simulink model "long_model72423"  (R2023a)
settings: Solver=VariableStepAuto  StartTime=0.0  StopTime=600  RelTol=1e-3
undefined symbols (not defined in the file or in its folder): A_f, brakeTime, breakStrength, C_alpha, C_d, C_rr, C_s, eta_t, g, headWind, headWindTime, I_w, Im, k, l_f, l_r, lambda_f, lambda_t, M, Meq, motorDecrease, motorDecreaseTime, motorIncrease, motorIncreaseTime, motorStart, motorStartTime, mu, R_w, rho, roadSlopeTime, Vstart
libraries: simulink x1
settings Model: Creator=Samsung  LastModifiedBy=brianlesko
settings SolverCC: AlgebraicLoopSolver=TrustRegion
settings DataIOCC: ReturnWorkspaceOutputs=off
settings OptimizationCC: ReuseModelBlockBuffer=off
settings DebuggingCC: UnconnectedInputMsg=warning  UnconnectedOutputMsg=warning  UnconnectedLineMsg=warning  ArithmeticOperatorsInVariantConditions=warning
settings ModelReferenceCC: EnableRefExpFcnMdlSchedulingChecks=on
settings SFSimCC: SimUseLocalCustomCode=off  CustomCodeUndefinedFunction=UseInterfaceOnly
settings RTWCC: RTWUseLocalCustomCode=off
settings CodeAppCC: StateflowObjectComments=on

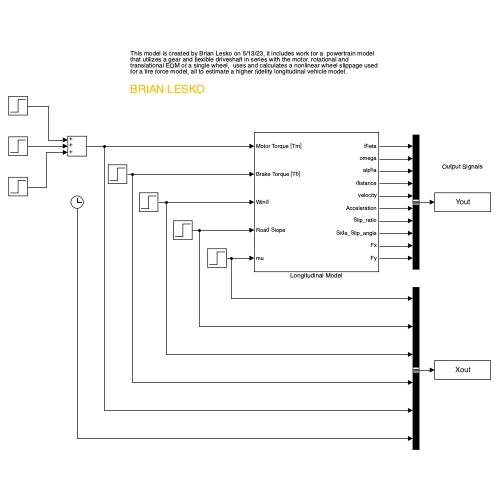
[thumbnail: Simulink's stored preview of the top-level diagram]
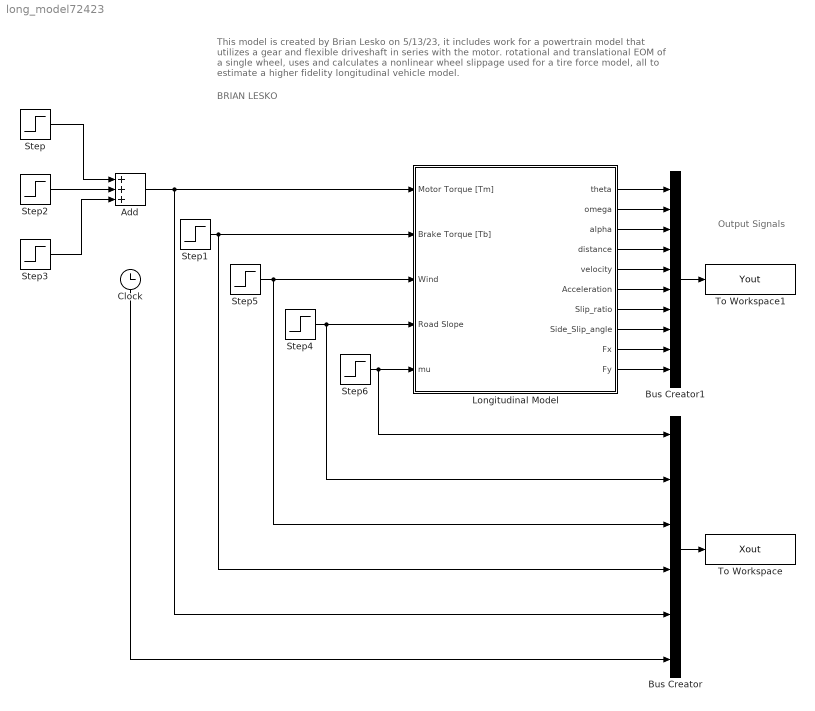
== system long_model72423 ==
  note: BRIAN LESKO
  note: This model is created by Brian Lesko on 5/13/23, it includes work for a powertrain model that utilizes a gear and flexible driveshaft in series with the motor. rotational and translational EOM of a single wheel, uses and calculates a nonlinear wheel slippage used for a tire force model, all to estimate a higher fidelity longitudinal vehicle model.
  note: Output Signals
  Add : Sum  Inputs=+++
  Bus Creator : BusCreator  Inputs=6
  Bus Creator1 : BusCreator  Inputs=10
  Clock : Clock
  Longitudinal Model : Subsystem
  Step : Step  Time=motorStartTime  After=motorStart  SampleTime=0
  Step1 : Step  Time=brakeTime  After=breakStrength  SampleTime=0
  Step2 : Step  Time=motorIncreaseTime  After=motorIncrease  SampleTime=0
  Step3 : Step  Time=motorDecreaseTime  After=-motorDecrease  SampleTime=0
  Step4 : Step  Time=roadSlopeTime  After=roadSlopeTime  SampleTime=0
  Step5 : Step  Time=headWindTime  After=headWind  SampleTime=0
  Step6 : Step  Time=0  Before=mu  After=mu  SampleTime=0
  To Workspace : ToWorkspace  VariableName=Xout  SampleTime=-1
  To Workspace1 : ToWorkspace  VariableName=Yout  SampleTime=-1
  wires:
  Step1/1 -> Longitudinal Model/2(Brake Torque [Tb]), Bus Creator/4
  Add/1 -> Bus Creator/5, Longitudinal Model/1(Motor Torque [Tm])
  Step2/1 -> Add/2
  Step3/1 -> Add/3
  Step/1 -> Add/1
  Step5/1 -> Bus Creator/3, Longitudinal Model/3(Wind)
  Step4/1 -> Bus Creator/2, Longitudinal Model/4(Road Slope)
  Step6/1 -> Bus Creator/1, Longitudinal Model/5(mu)
  Bus Creator/1 -> To Workspace/1
  Clock/1 -> Bus Creator/6
  Longitudinal Model/1(theta) -> Bus Creator1/1
  Longitudinal Model/2(omega) -> Bus Creator1/2
  Longitudinal Model/3(alpha) -> Bus Creator1/3
  Longitudinal Model/4(distance) -> Bus Creator1/4
  Longitudinal Model/5(velocity) -> Bus Creator1/5
  Longitudinal Model/6(Acceleration) -> Bus Creator1/6
  Longitudinal Model/7(Slip_ratio) -> Bus Creator1/7
  Longitudinal Model/8(Side_Slip_angle) -> Bus Creator1/8
  Longitudinal Model/9(Fx) -> Bus Creator1/9
  Longitudinal Model/10(Fy) -> Bus Creator1/10
  Bus Creator1/1 -> To Workspace1/1

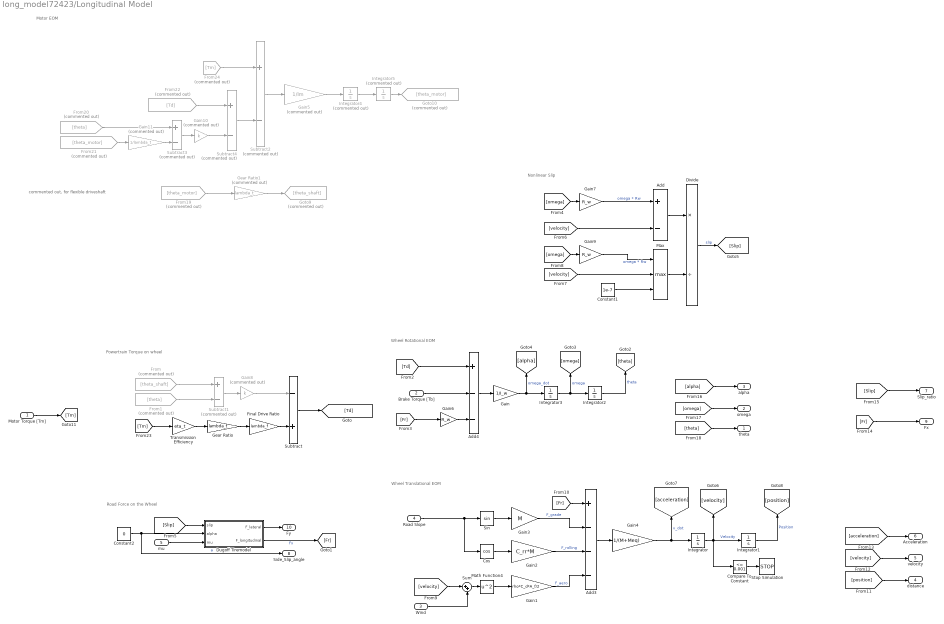
== system long_model72423/Longitudinal Model ==
  note: commented out, for flexible driveshaft
  note: Motor EOM
  note: Road Force on the Wheel
  note: Wheel Translational EOM
  note: Nonlinear Slip
  note: Wheel Rotational EOM
  note: Powertrain Torque on wheel
  Motor Torque [Tm] : Inport
  Brake Torque [Tb] : Inport  Port=2
  Wind : Inport  Port=3
  Road Slope : Inport  Port=4
  mu : Inport  Port=5
  Add : Sum  Inputs=+-
  Add3 : Sum  Inputs=+---
  Add4 : Sum  Inputs=+--
  Compare To Constant : simulink/Logic and Bit Operations/Compare To Constant  relop=<=  const=0.001  OutDataTypeStr=boolean
  Constant1 : Constant  Value=1e-7
  Constant2 : Constant  Value=0
  Cos : Trigonometry  Operator=cos
  Divide : Product  Inputs=*/
  Dugoff Tiremodel : Subsystem
  Final Drive Ratio : Gain  Gain=lambda_f
  From : From  Commented=on  GotoTag=theta_shaft
  From1 : From  Commented=on  GotoTag=theta
  From19 : From  Commented=on  GotoTag=theta_motor
  From20 : From  Commented=on  GotoTag=theta
  From21 : From  Commented=on  GotoTag=theta_motor
  From22 : From  Commented=on  GotoTag=Td
  From24 : From  Commented=on  GotoTag=Tm
  Gain : Gain  Gain=1/I_w
  Gain1 : Gain  Gain=rho*C_d*A_f/2
  Gain10 : Gain  Commented=on  Gain=k
  Gain11 : Gain  Commented=on  Gain=1/lambda_t
  Gain2 : Gain  Gain=C_rr*M
  Gain3 : Gain  Gain=M
  Gain4 : Gain  Gain=1/(M+Meq)
  Gain5 : Gain  Commented=on  Gain=1/Im
  Gain6 : Gain  Gain=R_w
  Gain7 : Gain  Gain=R_w
  Gain8 : Gain  Commented=on  Gain=k
  Gain9 : Gain  Gain=R_w
  Gear Ratio : Gain  Gain=lambda_t
  Gear Ratio1 : Gain  Commented=on  Gain=lambda_t
  Goto10 : Goto  Commented=on  GotoTag=theta_motor
  Goto9 : Goto  Commented=on  GotoTag=theta_shaft
  Integrator : Integrator  InitialCondition=Vstart  LimitOutput=on  LowerSaturationLimit=0
  Integrator1 : Integrator
  Integrator2 : Integrator  InitialCondition=1
  Integrator3 : Integrator  InitialCondition=1
  Integrator4 : Integrator  Commented=on  InitialCondition=1
  Integrator5 : Integrator  Commented=on  InitialCondition=1
  Math Function4 : Math  Operator=square  SignedPower=on
  Max : MinMax  Function=max  Inputs=3
  Sin : Trigonometry
  Stop Simulation : Stop
  Subtract : Sum  Inputs=-+
  Subtract{1..4} (4 alike) : Sum  Commented=on  Inputs=+-
  Sum : Sum  Inputs=|++
  Transmission Efficiency : Gain  Gain=eta_t
  theta : Outport  VectorParamsAs1DForOutWhenUnconnected=off
  omega : Outport  Port=2  VectorParamsAs1DForOutWhenUnconnected=off
  alpha : Outport  Port=3  VectorParamsAs1DForOutWhenUnconnected=off
  distance : Outport  Port=4  VectorParamsAs1DForOutWhenUnconnected=off
  velocity : Outport  Port=5  VectorParamsAs1DForOutWhenUnconnected=off
  Acceleration : Outport  Port=6  VectorParamsAs1DForOutWhenUnconnected=off
  Slip_ratio : Outport  Port=7
  Side_Slip_angle : Outport  Port=8
  Fx : Outport  Port=9
  Fy : Outport  Port=10
  wires:
  Integrator/1 -> Compare To Constant/1, Integrator1/1, [velocity]  "Velocity"
  Brake Torque [Tb]/1 -> Add4/2
  Compare To Constant/1 -> Stop Simulation/1
  Road Slope/1 -> Cos/1, Sin/1
  Sin/1 -> Gain3/1
  Gain2/1 -> Add3/3  "F_rolling"
  Add3/1 -> Gain4/1
  Constant2/1 -> Side_Slip_angle/1, Dugoff Tiremodel/2(alpha)  "a"
  Wind/1 -> Sum/2
  Gain7/1 -> Add/1  "omega * Rw"
  Cos/1 -> Gain2/1
  Gear Ratio/1 -> Final Drive Ratio/1
  Constant1/1 -> Max/3
  Gain/1 -> Integrator3/1, [alpha]  "omega_dot"
  Max/1 -> Divide/2
  Gain4/1 -> Integrator/1, [acceleration]  "v_dot"
  Math Function4/1 -> Gain1/1
  Transmission Efficiency/1 -> Gear Ratio/1
  Integrator3/1 -> Integrator2/1, [omega]  "omega"
  Gain1/1 -> Add3/4  "F_aero"
  Dugoff Tiremodel/1(F_lateral) -> Fy/1
  Add4/1 -> Gain/1
  Add/1 -> Divide/1
  Gain3/1 -> Add3/2  "F_grade"
  Gain6/1 -> Add4/3
  Dugoff Tiremodel/2(F_longitudinal) -> [Fr]  "Fx"
  Sum/1 -> Math Function4/1
  mu/1 -> Dugoff Tiremodel/3(mu)
  Subtract/1 -> [Td]
  From/1 -> Subtract1/1
  From1/1 -> Subtract1/2
  Subtract1/1 -> Gain8/1
  Final Drive Ratio/1 -> Subtract/2
  Gain8/1 -> Subtract/1
  [Td] -> Add4/1
  [Fr] -> Gain6/1
  Integrator2/1 -> [theta]  "theta"
  [omega] -> Gain7/1
  Divide/1 -> [Slip]  "slip"
  [Slip] -> Dugoff Tiremodel/1(slip)
  [velocity] -> Add/2
  [velocity] -> Max/2
  [omega] -> Gain9/1
  Gain9/1 -> Max/1  "omega * Rw"
  [velocity] -> Sum/1
  [Fr] -> Add3/1
  Integrator1/1 -> [position]  "Position"
  [position] -> distance/1
  [velocity] -> velocity/1
  [acceleration] -> Acceleration/1
  [Fr] -> Fx/1
  [Slip] -> Slip_ratio/1
  [alpha] -> alpha/1
  [omega] -> omega/1
  [theta] -> theta/1
  Gear Ratio1/1 -> Goto9/1
  From19/1 -> Gear Ratio1/1
  Integrator4/1 -> Integrator5/1
  Integrator5/1 -> Goto10/1
  Gain5/1 -> Integrator4/1
  From24/1 -> Subtract2/1
  Subtract2/1 -> Gain5/1
  Subtract3/1 -> Gain10/1
  From20/1 -> Subtract3/1
  Gain11/1 -> Subtract3/2
  From21/1 -> Gain11/1
  Subtract4/1 -> Subtract2/2
  Gain10/1 -> Subtract4/2
  From22/1 -> Subtract4/1
  Motor Torque [Tm]/1 -> [Tm]
  [Tm] -> Transmission Efficiency/1

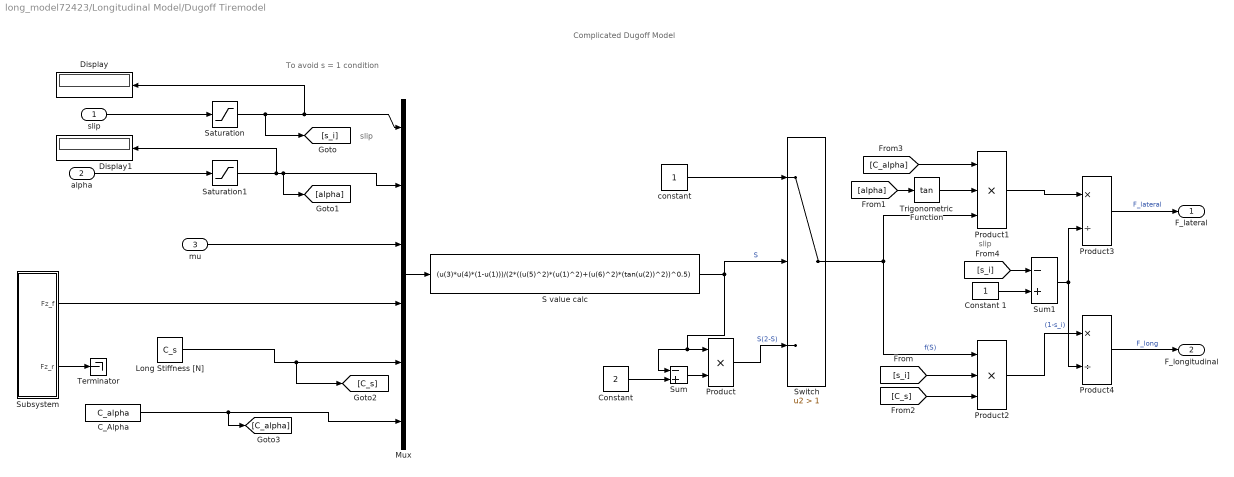
== system long_model72423/Longitudinal Model/Dugoff Tiremodel ==
  note: slip
  note: To avoid s = 1 condition
  note: Complicated Dugoff Model
  note: slip
  slip : Inport
  alpha : Inport  Port=2
  mu : Inport  Port=3
  C_Alpha : Constant  Value=C_alpha
  "Constant " : Constant  Value=2
  Constant 1 : Constant
  Display : Display
  Display1 : Display
  Long Stiffness [N] : Constant  Value=C_s
  Mux : Mux  Inputs=6
  Product : Product
  Product1 : Product  Inputs=3
  Product2 : Product  Inputs=3
  Product3 : Product  Inputs=*/
  Product4 : Product  Inputs=*/
  S value calc : Fcn  Expr=(u(3)*u(4)*(1-u(1)))/(2*((u(5)^2)*(u(1)^2)+(u(6)^2)*(tan(u(2))^2))^0.5)
  Saturation : Saturate  UpperLimit=0.999  LowerLimit=-1
  Saturation1 : Saturate  UpperLimit=20  LowerLimit=1e-4
  Subsystem : Subsystem
  Sum : Sum  Inputs=-+
  Sum1 : Sum  Inputs=-+
  Switch : Switch  Criteria=u2 > Threshold  Threshold=1  SaturateOnIntegerOverflow=off  InputSameDT=off
  Terminator : Terminator
  Trigonometric Function : Trigonometry  Operator=tan
  constant : Constant
  F_lateral : Outport  VectorParamsAs1DForOutWhenUnconnected=off
  F_longitudinal : Outport  Port=2  VectorParamsAs1DForOutWhenUnconnected=off
  wires:
  Switch/1 -> Product2/1, Product1/3  "f(S)"
  [s_i] -> Sum1/1
  Trigonometric Function/1 -> Product1/2
  Sum1/1 -> Product3/2, Product4/2  "(1-s_i)"
  [alpha] -> Trigonometric Function/1
  [C_alpha] -> Product1/1
  [s_i] -> Product2/2
  [C_s] -> Product2/3
  Product2/1 -> Product4/1
  Product1/1 -> Product3/1
  Product4/1 -> F_longitudinal/1  "F_long"
  Constant 1/1 -> Sum1/2
  Product3/1 -> F_lateral/1  "F_lateral"
  Sum/1 -> Product/2
  Subsystem/1(Fz_f) -> Mux/4
  "Constant "/1 -> Sum/2
  Saturation/1 -> Display/1, Mux/1, [s_i]
  mu/1 -> Mux/3
  Mux/1 -> S value calc/1
  Long Stiffness [N]/1 -> [C_s], Mux/5
  S value calc/1 -> Switch/2, Product/1, Sum/1  "S"
  slip/1 -> Saturation/1
  alpha/1 -> Saturation1/1
  C_Alpha/1 -> [C_alpha], Mux/6
  Saturation1/1 -> Display1/1, [alpha], Mux/2
  constant/1 -> Switch/1
  Product/1 -> Switch/3  "S(2-S)"
  Subsystem/2(Fz_r) -> Terminator/1

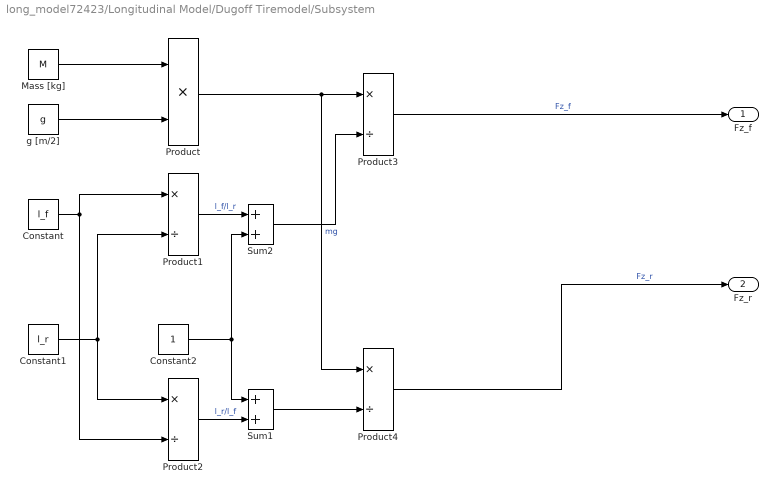
== system long_model72423/Longitudinal Model/Dugoff Tiremodel/Subsystem ==
  Constant : Constant  Value=l_f
  Constant1 : Constant  Value=l_r
  Constant2 : Constant
  Mass [kg] : Constant  Value=M
  Product : Product  Inputs=**
  Product{1..4} (4 alike) : Product  Inputs=*/
  Sum1 : Sum
  Sum2 : Sum
  g [m/2] : Constant  Value=g
  Fz_f : Outport  VectorParamsAs1DForOutWhenUnconnected=off
  Fz_r : Outport  Port=2  VectorParamsAs1DForOutWhenUnconnected=off
  wires:
  Sum2/1 -> Product3/2
  Product2/1 -> Sum1/2  "l_r/l_f"
  Sum1/1 -> Product4/2
  Product4/1 -> Fz_r/1  "Fz_r"
  Constant1/1 -> Product2/1, Product1/2
  Product/1 -> Product3/1, Product4/1  "mg"
  Constant/1 -> Product1/1, Product2/2
  Constant2/1 -> Sum1/1, Sum2/2
  Product1/1 -> Sum2/1  "l_f/l_r"
  Product3/1 -> Fz_f/1  "Fz_f"
  Mass [kg]/1 -> Product/1
  g [m/2]/1 -> Product/2
